simulink model "simulation_poleplacement_azioneintegrale_WP2_NL"  (R2023b)
settings: Solver=VariableStepAuto  StartTime=0.0  StopTime=20  RelTol=1e-3
values from neighbouring files (symbols this model uses):
  K = [k1 k2 ki]    [WP2.m]
  r = pi    (= 3.14159265359)    [WP2.m]
settings Model: Creator=miche  LastModifiedBy=miche

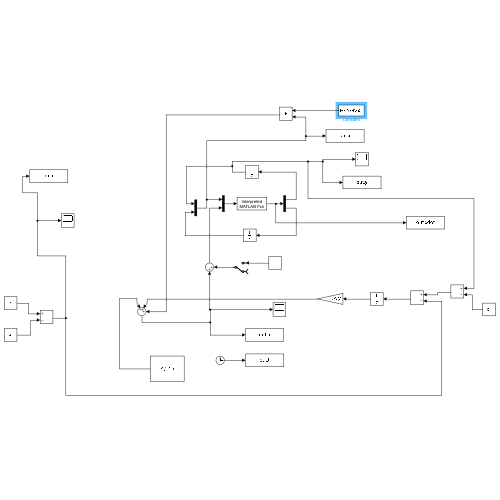
[thumbnail: Simulink's stored preview of the top-level diagram]
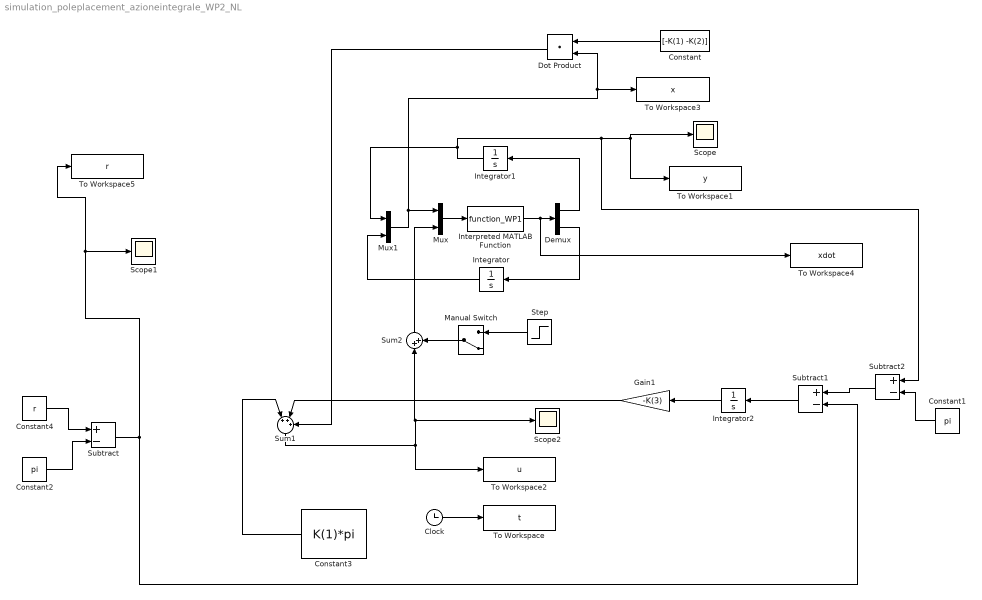
== system simulation_poleplacement_azioneintegrale_WP2_NL ==
  Clock : Clock
  Constant : Constant  Value=[-K(1) -K(2)]
  Constant1 : Constant  Value=pi
  Constant2 : Constant  Value=pi
  Constant3 : Constant  Value=K(1)*pi
  Constant4 : Constant  Value=r
  Demux : Demux  Outputs=2
  Dot Product : DotProduct  OutDataTypeStr=Inherit: Inherit via internal rule
  Gain1 : Gain  Gain=-K(3)
  Integrator : Integrator
  Integrator1 : Integrator
  Integrator2 : Integrator
  Interpreted MATLAB Function : MATLABFcn  MATLABFcn=function_WP1  OutputDimensions=2
  Manual Switch : ManualSwitch  CurrentSetting=0
  Mux : Mux  Inputs=2
  Mux1 : Mux  Inputs=2
  Scope : Scope
  Scope1 : Scope
  Scope2 : Scope
  Step : Step  Time=5  After=10000  SampleTime=0
  Subtract : Sum  Inputs=+-
  Subtract1 : Sum  Inputs=+-
  Subtract2 : Sum  Inputs=+-
  Sum1 : Sum  Inputs=|+++
  Sum2 : Sum  Inputs=|++
  To Workspace : ToWorkspace  VariableName=t  SampleTime=-1
  To Workspace1 : ToWorkspace  VariableName=y  SampleTime=-1
  To Workspace2 : ToWorkspace  VariableName=u  SampleTime=-1
  To Workspace3 : ToWorkspace  VariableName=x  SampleTime=-1
  To Workspace4 : ToWorkspace  VariableName=xdot  SampleTime=-1
  To Workspace5 : ToWorkspace  VariableName=r  SampleTime=-1
  wires:
  Demux/1 -> Integrator1/1
  Dot Product/1 -> Sum1/3
  Constant3/1 -> Sum1/1
  Mux/1 -> Interpreted MATLAB Function/1
  Constant2/1 -> Subtract/2
  Mux1/1 -> Dot Product/2, To Workspace3/1, Mux/1
  Constant4/1 -> Subtract/1
  Integrator/1 -> Mux1/2
  Sum1/1 -> Scope2/1, Sum2/1, To Workspace2/1
  Clock/1 -> To Workspace/1
  Constant/1 -> Dot Product/1
  Integrator1/1 -> Subtract2/1, Scope/1, To Workspace1/1, Mux1/1
  Interpreted MATLAB Function/1 -> To Workspace4/1, Demux/1
  Demux/2 -> Integrator/1
  Subtract/1 -> Scope1/1, To Workspace5/1, Subtract1/2
  Integrator2/1 -> Gain1/1
  Subtract1/1 -> Integrator2/1
  Subtract2/1 -> Subtract1/1
  Gain1/1 -> Sum1/2
  Constant1/1 -> Subtract2/2
  Step/1 -> Manual Switch/1
  Manual Switch/1 -> Sum2/2
  Sum2/1 -> Mux/2
